simulink model "spiBitbangSimulink_v3"  (R2013b)
settings: Solver=ode3  StartTime=0.0  StopTime=5e-3  FixedStep=sampleTime  MaxStep=MaxStepSize  RelTol=1e-3
undefined symbols (not defined in the file or in its folder): High, peri, periSam, pulse, pulseSam, sampleTime
libraries: dspswit3 x5, simulink x3, simulink_extras x1
settings Model: ExtModeTrigDuration=100  Creator=mainster  LastModifiedBy=mainster
settings OptimizationCC: OptimizeModelRefInitCode=on  LifeSpan=1
settings DebuggingCC: SolverPrmCheckMsg=none
settings HardwareCC: ProdLargestAtomicInteger=Long  ProdLargestAtomicFloat=Double  ProdEndianess=LittleEndian  ProdHWDeviceType=ARM Compatible->ARM Cortex
settings RTWCC: SystemTargetFile=realtime.tlc  GenerateMakefile=off  TemplateMakefile=realtime.tmf  Description=Run on Target Hardware  RTWVerbose=off  ProcessScript=realtime_make_rtw_hook
settings STFCustomTargetCC: TargetLibSuffix=.a  GenerateSampleERTMain=on  ERTCustomFileBanners=on  SupportNonInlinedSFcns=off  SupportVariableSizeSignals=on  MATLABClassNameForMDSCustomization=Simulink.SoftwareTarget.ERTCustomization  GRTInterface=off  SystemTargetFile=realtime.tlc
settings ERTTargetCC: CodeReplacementLibrary=ANSI_C  GenerateSampleERTMain=on  ParMdlRefBuildCompliant=off  CompOptLevelCompliant=off  ConcurrentExecutionCompliant=off  CombineOutputUpdateFcns=off  ERTFirstTimeCompliant=off  SupportContinuousTime=on  SupportVariableSizeSignals=on  ModelStepFunctionPrototypeControlCompliant=off  CPPClassGenCompliant=off  ExtModeMexArgs='192.168.2.111' 0 17725  InlinedParameterPlacement=NonHierarchical  ERTSrcFileBannerTemplate=realtime_code_template.cgt  ERTHdrFileBannerTemplate=realtime_code_template.cgt  ERTDataSrcFileTemplate=realtime_code_template.cgt  ERTDataHdrFileTemplate=realtime_code_template.cgt  ERTCustomFileTemplate=realtime_file_process.tlc

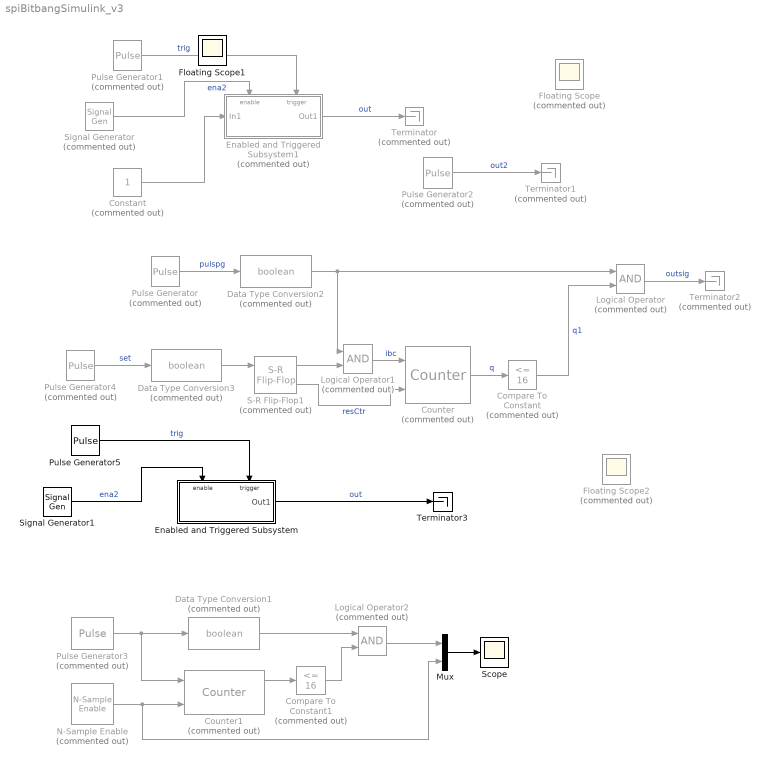
== system spiBitbangSimulink_v3 ==
  Compare To Constant : simulink/Logic and Bit Operations/Compare To Constant  Commented=on  relop=<=  const=16  OutDataTypeStr=boolean
  Compare To Constant1 : simulink/Logic and Bit Operations/Compare To Constant  Commented=on  relop=<=  const=16  OutDataTypeStr=boolean
  Constant : Constant  Commented=on  OutDataTypeStr=double  SampleTime=sampleTime
  Counter : dspswit3/Counter  Commented=on  Direction=Up  CountEvent=Rising edge  CounterSize=8 bits  MaxCount=255  InitialCount=0  Output=Count  HitValue=32  ResetInput=on  SamplesPerFrame=1  Ts=1  CntDtype=uint8  HitDtype=Logical
  Counter1 : dspswit3/Counter  Commented=on  Direction=Down  CountEvent=Rising edge  CounterSize=User defined  MaxCount=20  InitialCount=0  Output=Count and Hit  HitValue=4  ResetInput=on  SamplesPerFrame=1  Ts=1  CntDtype=double  HitDtype=Logical
  Data Type Conversion1 : DataTypeConversion  Commented=on  OutDataTypeStr=boolean
  Data Type Conversion2 : DataTypeConversion  Commented=on  OutDataTypeStr=boolean
  Data Type Conversion3 : DataTypeConversion  Commented=on  OutDataTypeStr=boolean
  Enabled and Triggered Subsystem : Subsystem  TreatAsAtomicUnit=on
  Enabled and Triggered Subsystem1 : Subsystem  Commented=on  TreatAsAtomicUnit=on
  Floating Scope : Scope  Commented=on  NumInputPorts=3
      settings: Floating=on  TimeRange=0.005  YMin=-0.1~-0.1~-0.1  YMax=1.1~1.1~1.1
  Floating Scope2 : Scope  Commented=on  NumInputPorts=3
      settings: Floating=on  TimeRange=0.005  YMin=-0.1~-0.1~-0.1  YMax=1.1~1.1~1.1
  Logical Operator : Logic  Commented=on  AllPortsSameDT=off  OutDataTypeStr=boolean
  Logical Operator1 : Logic  Commented=on  AllPortsSameDT=off  OutDataTypeStr=boolean
  Logical Operator2 : Logic  Commented=on  AllPortsSameDT=off  OutDataTypeStr=boolean
  Mux : Mux  Inputs=2
  N-Sample Enable : dspswit3/N-Sample Enable  Commented=on  N=250  ActiveLevel=High (1)  reset=off  TriggerType=Rising edge  Ts=sampleTime  DataType=Logical
  Pulse Generator : DiscretePulseGenerator  Commented=on  Period=83  PulseWidth=25  SampleTime=sampleTime
  Pulse Generator1 : DiscretePulseGenerator  Commented=on  Period=200  PulseWidth=150  SampleTime=sampleTime
  Pulse Generator2 : DiscretePulseGenerator  Commented=on  Period=periSam  PulseWidth=pulseSam  SampleTime=-1
  Pulse Generator3 : DiscretePulseGenerator  Commented=on  Period=50  PulseWidth=25  SampleTime=sampleTime
  Pulse Generator4 : DiscretePulseGenerator  Commented=on  Period=100  PulseWidth=50  PhaseDelay=10  SampleTime=sampleTime
  Pulse Generator5 : DiscretePulseGenerator  Period=200  PulseWidth=150  SampleTime=sampleTime
  S-R Flip-Flop1 : simulink_extras/Flip Flops/S-R Flip-Flop  Commented=on  initial_condition=0
  Scope : Scope
      settings: SaveName=ScopeData2
  Signal Generator : SignalGenerator  Commented=on  WaveForm=square  Frequency=1e3
  Signal Generator1 : SignalGenerator  WaveForm=square  Frequency=1e3
  Terminator : Terminator  Commented=on
  Terminator1 : Terminator  Commented=on
  Terminator2 : Terminator  Commented=on
  Terminator3 : Terminator
  Floating Scope1 : Scope
      settings: Floating=on  SaveName=ScopeData3
  wires:
  Pulse Generator/1 -> Data Type Conversion2/1  "pulspg"
  Counter/1 -> Compare To Constant/1  "q"
  Compare To Constant/1 -> Logical Operator/2  "q1"
  S-R Flip-Flop1/1 -> Logical Operator1/2
  Logical Operator1/1 -> Counter/1  "ibc"
  Pulse Generator4/1 -> Data Type Conversion3/1  "set"
  S-R Flip-Flop1/2 -> Counter/2  "resCtr"
  Data Type Conversion2/1 -> Logical Operator1/1, Logical Operator/1
  Data Type Conversion3/1 -> S-R Flip-Flop1/1
  Enabled and Triggered Subsystem1/1(Out1) -> Terminator/1  "out"
  Pulse Generator1/1 -> Enabled and Triggered Subsystem1/Trigger  "trig"
  Signal Generator/1 -> Enabled and Triggered Subsystem1/Enable  "ena2"
  Pulse Generator2/1 -> Terminator1/1  "out2"
  Constant/1 -> Enabled and Triggered Subsystem1/1(In1)
  Logical Operator/1 -> Terminator2/1  "outsig"
  Pulse Generator3/1 -> Counter1/1, Data Type Conversion1/1
  N-Sample Enable/1 -> Counter1/2, Mux/2
  Data Type Conversion1/1 -> Logical Operator2/1
  Logical Operator2/1 -> Mux/1
  Mux/1 -> Scope/1
  Counter1/1 -> Compare To Constant1/1
  Compare To Constant1/1 -> Logical Operator2/2
  Enabled and Triggered Subsystem/1(Out1) -> Terminator3/1  "out"
  Pulse Generator5/1 -> Enabled and Triggered Subsystem/Trigger  "trig"
  Signal Generator1/1 -> Enabled and Triggered Subsystem/Enable  "ena2"

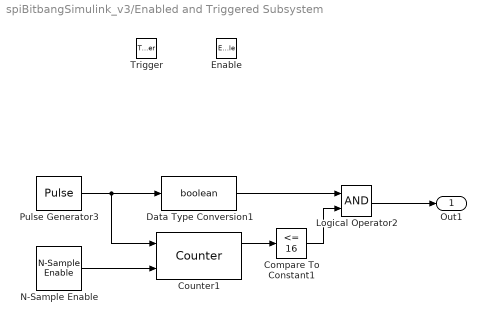
== system spiBitbangSimulink_v3/Enabled and Triggered Subsystem ==
  Enable : EnablePort
  Trigger : TriggerPort
  Compare To Constant1 : simulink/Logic and Bit Operations/Compare To Constant  relop=<=  const=16  OutDataTypeStr=boolean
  Counter1 : dspswit3/Counter  Direction=Down  CountEvent=Rising edge  CounterSize=User defined  MaxCount=20  InitialCount=0  Output=Count and Hit  HitValue=4  ResetInput=on  SamplesPerFrame=1  Ts=1  CntDtype=double  HitDtype=Logical
  Data Type Conversion1 : DataTypeConversion  OutDataTypeStr=boolean
  Logical Operator2 : Logic  AllPortsSameDT=off  OutDataTypeStr=boolean
  N-Sample Enable : dspswit3/N-Sample Enable  N=250  ActiveLevel=High (1)  reset=off  TriggerType=Rising edge  Ts=-1  DataType=Logical
  Pulse Generator3 : DiscretePulseGenerator  Period=50  PulseWidth=25  SampleTime=-1
  Out1 : Outport
  wires:
  Pulse Generator3/1 -> Counter1/1, Data Type Conversion1/1
  N-Sample Enable/1 -> Counter1/2
  Data Type Conversion1/1 -> Logical Operator2/1
  Counter1/1 -> Compare To Constant1/1
  Compare To Constant1/1 -> Logical Operator2/2
  Logical Operator2/1 -> Out1/1

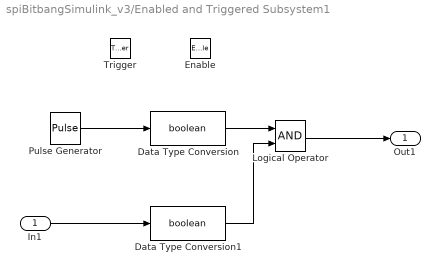
== system spiBitbangSimulink_v3/Enabled and Triggered Subsystem1 ==
  In1 : Inport
  Enable : EnablePort
  Trigger : TriggerPort
  Data Type Conversion : DataTypeConversion  OutDataTypeStr=boolean
  Data Type Conversion1 : DataTypeConversion  OutDataTypeStr=boolean
  Logical Operator : Logic  AllPortsSameDT=off  OutDataTypeStr=boolean
  Pulse Generator : DiscretePulseGenerator  PulseType=Time based  Period=peri  PulseWidth=pulse  SampleTime=-1
  Out1 : Outport
  wires:
  Logical Operator/1 -> Out1/1
  Pulse Generator/1 -> Data Type Conversion/1
  In1/1 -> Data Type Conversion1/1
  Data Type Conversion/1 -> Logical Operator/1
  Data Type Conversion1/1 -> Logical Operator/2
